simulink model "bullet_6dof"  (R2026a)
settings: Solver=VariableStepAuto
values from neighbouring files (symbols this model uses):
  g = 9.81    [bulletM2sim.m]
  m = 0.00985    [bulletM2sim.m]
settings Model: Creator=chris  LastModifiedBy=chris

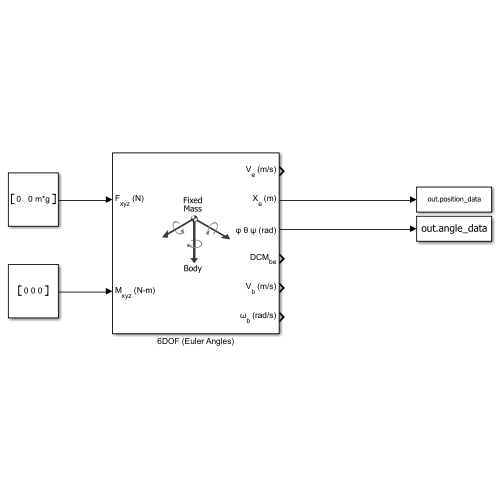
[thumbnail: Simulink's stored preview of the top-level diagram]
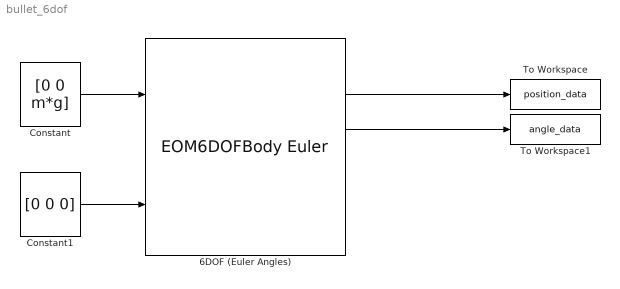
== system bullet_6dof ==
  6DOF (Euler Angles) : EOM6DOFBodyEuler  Vm_0=[750 0 0]  pm_0=[180000 * (2*pi/60) 0 0]
  Constant : Constant  Value=[0 0 m*g]
  Constant1 : Constant  Value=[0 0 0]
  To Workspace : ToWorkspace  VariableName=position_data  SaveFormat=Timeseries  SampleTime=-1
  To Workspace1 : ToWorkspace  VariableName=angle_data  SaveFormat=Timeseries  SampleTime=-1
  wires:
  6DOF (Euler Angles)/2 -> To Workspace/1
  6DOF (Euler Angles)/3 -> To Workspace1/1
  Constant/1 -> 6DOF (Euler Angles)/1
  Constant1/1 -> 6DOF (Euler Angles)/2
